simulink subsystem "AllControllers"  (R2020b)
settings: Solver=VariableStepAuto  StartTime=0.0  StopTime=10.0  RelTol=1e-3
values from neighbouring files (symbols this model uses):
  A = d_sys.A    [MPC_Init.m]    (also in init.m = [a11 a12 0 0;     a21 a22 0 0;     0 1 0 0;     v ls v 0])
  B = d_sys.B    [MPC_Init.m]    (also in init.m = [2*cf/(m*v) 0; 2*lf*cf/iz 0; 0 -v ;0  0])
  C = d_sys.C    [MPC_Init.m]    (also in init.m = [0 0 1 0; 0 0 0 1])
  K = place(A,B,kp)    [init.m]
  L = place(A',C',kl)    [init.m]
  Ts = 0.1    [MPC_Init.m]
undefined symbols (not defined in the file or in its folder): DiscIntNeverNeededParam, lkasubsystem_1_data, PredictionHorizon
libraries: mpclib x1, simulink x1, mpcadaslib x1, pid_lib x1
settings Model: Creator=Stage  LastModifiedBy=Stage

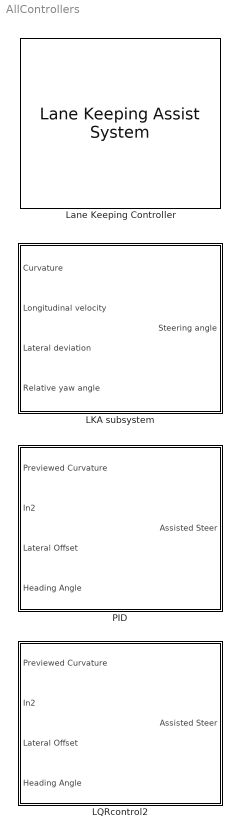
== system AllControllers ==
  LKA subsystem : Subsystem
  LQRcontrol2 : Subsystem
  Lane Keeping Controller : mpcadaslib/Lane Keeping Assist System  ModelType=Use vehicle parameters  VehicleMass=m  VehicleYawInertia=Iz  LengthToFront=lf  LengthToRear=lr  FrontTireStiffness=Cf  RearTireStiffness=Cr  EgoModelMatrixA=[-4.4021 ,-12.4603;1.3913,-5.1868]  EgoModelMatrixB=[24.1270;15.8609]  EgoModelMatrixC=[1,0;0,1]  InitialLongVel=v0_ego  TransportLag=0  MinSteering=-0.5  umin_ext=off  MaxSteering=0.5  umax_ext=off  Ts=Ts  PredictionHorizon=PredictionHorizon  ControllerBehavior=0.200  suboptimal=off  maxiter=10  datatypeopt=single  optmode=off  trackmode=off
      settings: SourceProductBaseCode=MP
  PID : Subsystem

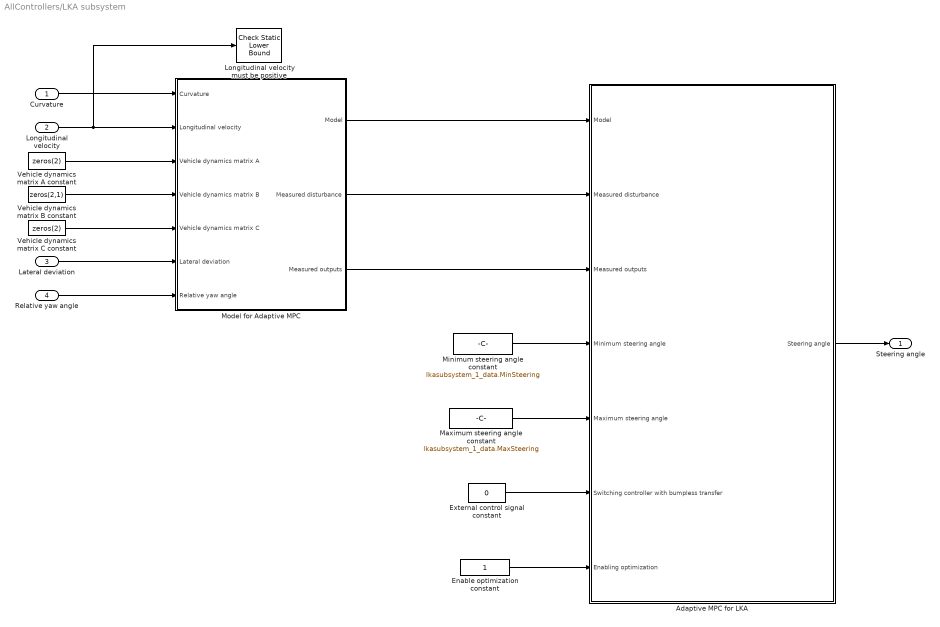
== system AllControllers/LKA subsystem ==
  Curvature : Inport
  Longitudinal velocity : Inport  Port=2
  Lateral deviation : Inport  Port=3
  Relative yaw angle : Inport  Port=4
  Adaptive MPC for LKA : Subsystem
  Enable optimization constant : Constant  OutDataTypeStr=lkasubsystem_1_data.DataType
  External control signal constant : Constant  Value=0  OutDataTypeStr=lkasubsystem_1_data.DataType
  Longitudinal velocity must be positive : simulink/Model Verification/Check Static  Lower Bound  Description=0 < u  min=0  min_included=off  enabled=on  stopWhenAssertionFail=on  export=off  icon=graphic
  Maximum steering angle constant : Constant  Value=lkasubsystem_1_data.MaxSteering  OutDataTypeStr=lkasubsystem_1_data.DataType
  Minimum steering angle constant : Constant  Value=lkasubsystem_1_data.MinSteering  OutDataTypeStr=lkasubsystem_1_data.DataType
  Model for Adaptive MPC : Subsystem
  Vehicle dynamics matrix A constant : Constant  Value=zeros(2)  OutDataTypeStr=lkasubsystem_1_data.DataType
  Vehicle dynamics matrix B constant : Constant  Value=zeros(2,1)  OutDataTypeStr=lkasubsystem_1_data.DataType
  Vehicle dynamics matrix C constant : Constant  Value=zeros(2)  OutDataTypeStr=lkasubsystem_1_data.DataType
  Steering angle : Outport  VectorParamsAs1DForOutWhenUnconnected=off
  wires:
  Longitudinal velocity/1 -> Longitudinal velocity must be positive/1, Model for Adaptive MPC/2(Longitudinal velocity)
  Curvature/1 -> Model for Adaptive MPC/1(Curvature)
  Model for Adaptive MPC/1(Model) -> Adaptive MPC for LKA/1(Model)
  Adaptive MPC for LKA/1(Steering angle) -> Steering angle/1
  Model for Adaptive MPC/2(Measured disturbance) -> Adaptive MPC for LKA/2(Measured disturbance)
  Enable optimization constant/1 -> Adaptive MPC for LKA/7(Enabling optimization)
  External control signal constant/1 -> Adaptive MPC for LKA/6(Switching controller with bumpless transfer)
  Minimum steering angle constant/1 -> Adaptive MPC for LKA/4(Minimum steering angle)
  Maximum steering angle constant/1 -> Adaptive MPC for LKA/5(Maximum steering angle)
  Model for Adaptive MPC/3(Measured outputs) -> Adaptive MPC for LKA/3(Measured outputs)
  Lateral deviation/1 -> Model for Adaptive MPC/6(Lateral deviation)
  Relative yaw angle/1 -> Model for Adaptive MPC/7(Relative yaw angle)
  Vehicle dynamics matrix A constant/1 -> Model for Adaptive MPC/3(Vehicle dynamics matrix A)
  Vehicle dynamics matrix B constant/1 -> Model for Adaptive MPC/4(Vehicle dynamics matrix B)
  Vehicle dynamics matrix C constant/1 -> Model for Adaptive MPC/5(Vehicle dynamics matrix C)

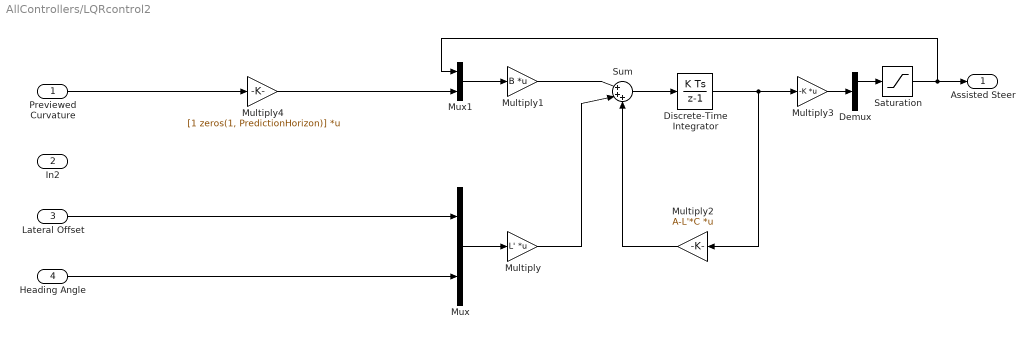
== system AllControllers/LQRcontrol2 ==
  Previewed Curvature : Inport
  In2 : Inport  Port=2
  Lateral Offset : Inport  Port=3
  Heading Angle : Inport  Port=4
  Demux : Demux  Outputs=2
  Discrete-Time Integrator : DiscreteIntegrator  SampleTime=-1  ICPrevOutput=DiscIntNeverNeededParam  ICPrevScaledInput=DiscIntNeverNeededParam
  Multiply : Gain  Gain=L'  Multiplication=Matrix(K*u) (u vector)
  Multiply1 : Gain  Gain=B  Multiplication=Matrix(K*u) (u vector)
  Multiply2 : Gain  Gain=A-L'*C  Multiplication=Matrix(K*u) (u vector)
  Multiply3 : Gain  Gain=-K  Multiplication=Matrix(K*u) (u vector)
  Multiply4 : Gain  Gain=[1 zeros(1, PredictionHorizon)]  Multiplication=Matrix(K*u) (u vector)
  Mux : Mux  Inputs=2
  Mux1 : Mux  Inputs=2
  Saturation : Saturate  UpperLimit=0.2  LowerLimit=-0.2
  Sum : Sum  Inputs=|+++
  Assisted Steer : Outport
  wires:
  Heading Angle/1 -> Mux/2
  Lateral Offset/1 -> Mux/1
  Mux/1 -> Multiply/1
  Demux/1 -> Saturation/1
  Previewed Curvature/1 -> Multiply4/1
  Multiply4/1 -> Mux1/2
  Mux1/1 -> Multiply1/1
  Multiply1/1 -> Sum/1
  Multiply/1 -> Sum/2
  Sum/1 -> Discrete-Time Integrator/1
  Discrete-Time Integrator/1 -> Multiply2/1, Multiply3/1
  Multiply2/1 -> Sum/3
  Multiply3/1 -> Demux/1
  Saturation/1 -> Assisted Steer/1, Mux1/1

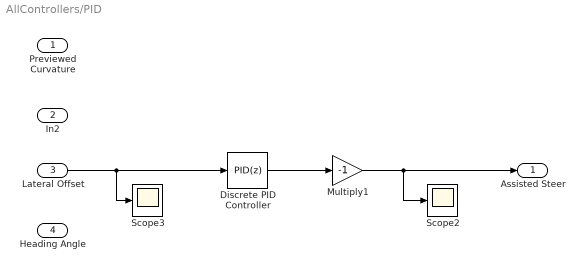
== system AllControllers/PID ==
  Previewed Curvature : Inport
  In2 : Inport  Port=2
  Lateral Offset : Inport  Port=3
  Heading Angle : Inport  Port=4
  Discrete PID Controller : pid_lib/PID Controller  Controller=PID  Form=Parallel  TimeDomain=Discrete-time  UseExternalTs=off  SampleTime=-1  IntegratorMethod=Forward Euler  FilterMethod=Forward Euler  ControllerParametersSource=internal  P=0.5  I=0.05  D=0.08  UseFilter=off  N=100  TunerSelectOption=Transfer Function Based (PID Tuner App)  InitialConditionSource=internal  InitialConditionForIntegrator=0  InitialConditionForFilter=0  DifferentiatorICPrevScaledInput=0  ExternalReset=none  TrackingMode=off  Kt=1  LimitOutput=off  SatLimitsSource=internal  UpperSaturationLimit=inf  LowerSaturationLimit=-inf  LinearizeAsGain=off  AntiWindupMode=none  Kb=1  POutMin=[]  POutMax=[]  IOutMin=[]  IOutMax=[]  DOutMin=[]  DOutMax=[]  NOutMin=[]  NOutMax=[]  SumOutMin=[]  SumOutMax=[]  SaturationOutMin=[]  SaturationOutMax=[]  PParamMin=[]  PParamMax=[]  IParamMin=[]  IParamMax=[]  DParamMin=[]  DParamMax=[]  NParamMin=[]  NParamMax=[]  KbParamMin=[]  KbParamMax=[]  KtParamMin=[]  KtParamMax=[]  KbOutMin=[]  KbOutMax=[]  KtOutMin=[]  KtOutMax=[]  IntegratorOutMin=[]  IntegratorOutMax=[]  FilterOutMin=[]  FilterOutMax=[]  SumI1OutMin=[]  SumI1OutMax=[]  SumI2OutMin=[]  SumI2OutMax=[]  SumI3OutMin=[]  SumI3OutMax=[]  SumI4OutMin=[]  SumI4OutMax=[]  SumDOutMin=[]  SumDOutMax=[]  DifferentiatorOutMin=[]  DifferentiatorOutMax=[]  FilterDiffOutCoefMin=[]  FilterDiffOutCoefMax=[]  ReciprocalOutMin=[]  ReciprocalOutMax=[]  SumDenOutMin=[]  SumDenOutMax=[]  SumNumOutMin=[]  SumNumOutMax=[]  DivideOutMin=[]  DivideOutMax=[]  UdiffTsProdOutMin=[]  UdiffTsProdOutMax=[]  NTsProdOutMin=[]  NTsProdOutMax=[]  UintegralTsProdOutMin=[]  UintegralTsProdOutMax=[]  UngainTsProdOutMin=[]  UngainTsProdOutMax=[]  IntegratorContinuousStateAttributes=''  IntegratorStateMustResolveToSignalObject=off  IntegratorRTWStateStorageClass=Auto  FilterContinuousStateAttributes=''  FilterStateMustResolveToSignalObject=off  FilterRTWStateStorageClass=Auto  ParallelPVariant=InternalParameters  IdealPVariant=Disabled  IVariant=InternalParameters  DVariant=InternalParameters  IntegratorVariant=Discrete  SatVariant=Disabled  AWVariant=Passthrough  PCopyVariant=Disabled  TRVariant=Disabled  FdbkBlocksVariant=Forward  IdealPFdbkVariant=Disabled  SatFdbkVariant=Disabled  DerivativeFilterVariant=Differentiator  NVariant=Passthrough  NCopyVariant=Disabled_SignalSpec  FilterICVariant=InternalICsDifferentiator  IntegratorICVariant=InternalICs  ExternalResetVariant=Disabled  TRSumVariant=Passthrough  SumFdbkVariant=Disabled  SumVariant=Sum_PID  TsampFilterVariant=InternalTs  TsampNgainVariant=Passthrough  TsampIntegralVariant=Passthrough  ExternalSaturationOutDataTypeStr=Inherit: Same as second input
  Multiply1 : Gain  Gain=-1
  Scope2 : Scope
  Scope3 : Scope
  Assisted Steer : Outport
  wires:
  Lateral Offset/1 -> Scope3/1, Discrete PID Controller/1
  Discrete PID Controller/1 -> Multiply1/1
  Multiply1/1 -> Assisted Steer/1, Scope2/1

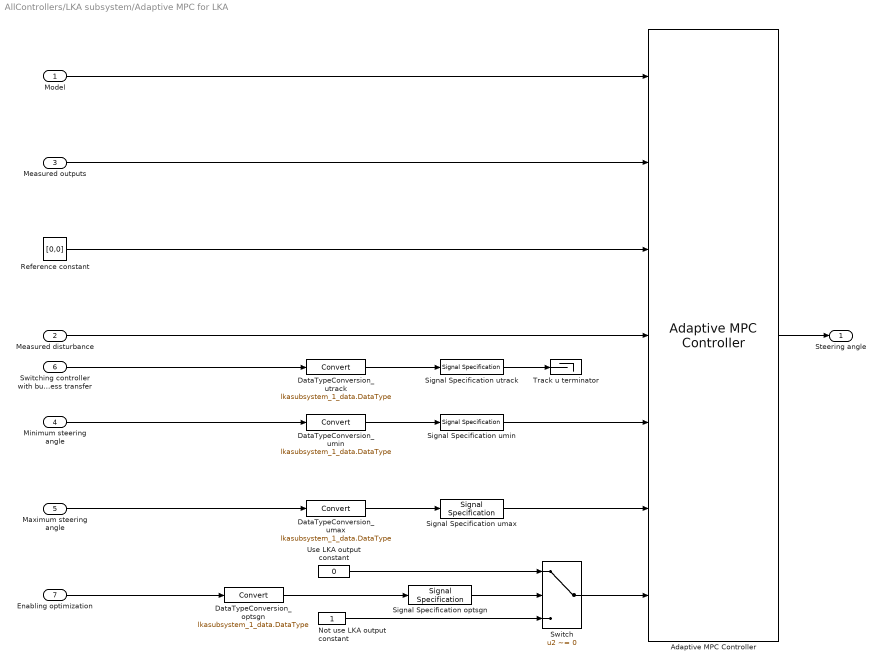
== system AllControllers/LKA subsystem/Adaptive MPC for LKA ==
  Model : Inport
  Measured disturbance : Inport  Port=2
  Measured outputs : Inport  Port=3
  Minimum steering angle : Inport  Port=4
  Maximum steering angle : Inport  Port=5
  Switching controller with bumpless transfer : Inport  Port=6
  Enabling optimization : Inport  Port=7
  Adaptive MPC Controller : mpclib/Adaptive MPC Controller  SCDEnableBlockLinearizationSpecification=on  mpcobj=lkasubsystem_1_data.Controller  enable_value=0  updateMPCinCallerWorkspace=off  md_inport=on  mv_inport=off  uref_inport=off  return_cost=off  return_mvseq=off  return_qpstatus=off  return_xseq=off  return_state=off  return_ovseq=off  state_inport=off  isltv_plant=off  umin_inport=on  umax_inport=on  ymin_inport=off  ymax_inport=off  cc_inport=off  ywt_inport=off  uwt_inport=off  duwt_inport=off  rhoeps_inport=off  pm_inport=off  MaximumP=10  HorizonChoice=FixedHorizon  BlockDataType=single  SampleTimeInherited=off  switch_inport=on
      settings: SourceProductName=Model Predictive Control Toolbox
  DataTypeConversion_optsgn : DataTypeConversion  OutDataTypeStr=lkasubsystem_1_data.DataType
  DataTypeConversion_umax : DataTypeConversion  OutDataTypeStr=lkasubsystem_1_data.DataType
  DataTypeConversion_umin : DataTypeConversion  OutDataTypeStr=lkasubsystem_1_data.DataType
  DataTypeConversion_utrack : DataTypeConversion  OutDataTypeStr=lkasubsystem_1_data.DataType
  Not use LKA output constant : Constant  OutDataTypeStr=lkasubsystem_1_data.DataType
  Reference constant : Constant  Value=[0,0]  VectorParams1D=off  OutDataTypeStr=lkasubsystem_1_data.DataType
  Signal Specification optsgn : SignalSpecification  Dimensions=1
  Signal Specification umax : SignalSpecification  Dimensions=1
  Signal Specification umin : SignalSpecification  Dimensions=1
  Signal Specification utrack : SignalSpecification  Dimensions=1
  Switch : Switch  Criteria=u2 ~= 0
  Track u terminator : Terminator
  Use LKA output constant : Constant  Value=0  OutDataTypeStr=lkasubsystem_1_data.DataType
  Steering angle : Outport  VectorParamsAs1DForOutWhenUnconnected=off
  wires:
  Not use LKA output constant/1 -> Switch/3
  DataTypeConversion_umin/1 -> Signal Specification umin/1
  Measured disturbance/1 -> Adaptive MPC Controller/4
  Switching controller with bumpless transfer/1 -> DataTypeConversion_utrack/1
  DataTypeConversion_umax/1 -> Signal Specification umax/1
  Use LKA output constant/1 -> Switch/1
  Adaptive MPC Controller/1 -> Steering angle/1
  DataTypeConversion_utrack/1 -> Signal Specification utrack/1
  DataTypeConversion_optsgn/1 -> Signal Specification optsgn/1
  Signal Specification optsgn/1 -> Switch/2
  Reference constant/1 -> Adaptive MPC Controller/3
  Switch/1 -> Adaptive MPC Controller/7
  Minimum steering angle/1 -> DataTypeConversion_umin/1
  Model/1 -> Adaptive MPC Controller/1
  Signal Specification umin/1 -> Adaptive MPC Controller/5
  Maximum steering angle/1 -> DataTypeConversion_umax/1
  Enabling optimization/1 -> DataTypeConversion_optsgn/1
  Measured outputs/1 -> Adaptive MPC Controller/2
  Signal Specification umax/1 -> Adaptive MPC Controller/6
  Signal Specification utrack/1 -> Track u terminator/1

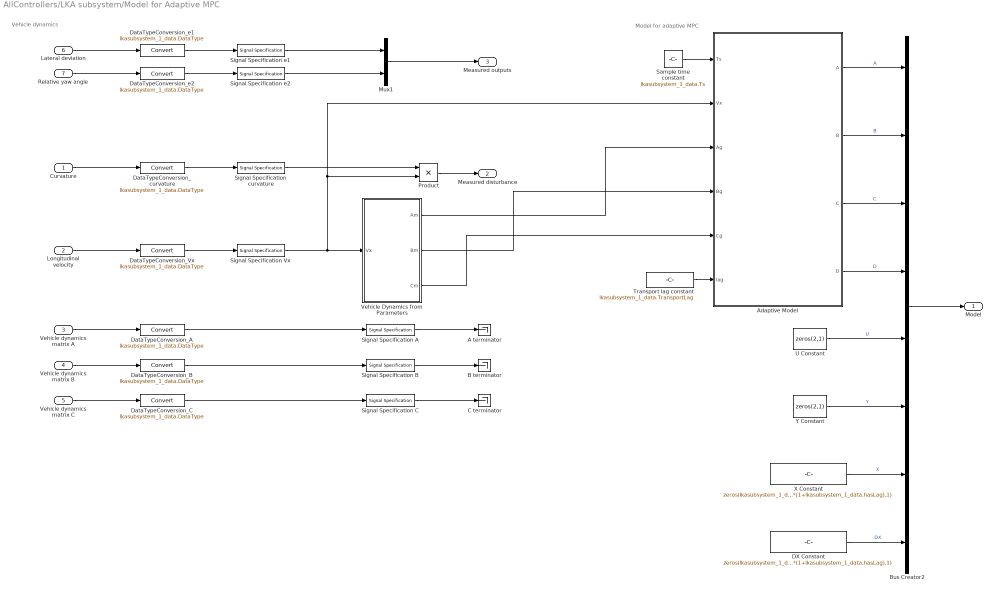
== system AllControllers/LKA subsystem/Model for Adaptive MPC ==
  note: Model for adaptive MPC
  note: Vehicle dynamics
  Curvature : Inport
  Longitudinal velocity : Inport  Port=2
  Vehicle dynamics matrix A : Inport  Port=3
  Vehicle dynamics matrix B : Inport  Port=4
  Vehicle dynamics matrix C : Inport  Port=5
  Lateral deviation : Inport  Port=6
  Relative yaw angle : Inport  Port=7
  A terminator : Terminator
  Adaptive Model : MATLAB Function  TreatAsAtomicUnit=on
  B terminator : Terminator
  Bus Creator2 : BusCreator  Inputs=8
  C terminator : Terminator
  DX Constant : Constant  Value=zeros(lkasubsystem_1_data.NumEgoStates+2*(1+lkasubsystem_1_data.hasLag),1)  VectorParams1D=off  OutDataTypeStr=lkasubsystem_1_data.DataType
  DataTypeConversion_A : DataTypeConversion  OutDataTypeStr=lkasubsystem_1_data.DataType
  DataTypeConversion_B : DataTypeConversion  OutDataTypeStr=lkasubsystem_1_data.DataType
  DataTypeConversion_C : DataTypeConversion  OutDataTypeStr=lkasubsystem_1_data.DataType
  DataTypeConversion_Vx : DataTypeConversion  OutDataTypeStr=lkasubsystem_1_data.DataType
  DataTypeConversion_curvature : DataTypeConversion  OutDataTypeStr=lkasubsystem_1_data.DataType
  DataTypeConversion_e1 : DataTypeConversion  OutDataTypeStr=lkasubsystem_1_data.DataType
  DataTypeConversion_e2 : DataTypeConversion  OutDataTypeStr=lkasubsystem_1_data.DataType
  Mux1 : Mux  Inputs=[1 1]
  Product : Product
  Sample time constant : Constant  Value=lkasubsystem_1_data.Ts  OutDataTypeStr=lkasubsystem_1_data.DataType
  Signal Specification A : SignalSpecification
  Signal Specification B : SignalSpecification
  Signal Specification C : SignalSpecification
  Signal Specification Vx : SignalSpecification  Dimensions=1
  Signal Specification curvature : SignalSpecification
  Signal Specification e1 : SignalSpecification  Dimensions=1
  Signal Specification e2 : SignalSpecification  Dimensions=1
  Transport lag constant : Constant  Value=lkasubsystem_1_data.TransportLag  OutDataTypeStr=lkasubsystem_1_data.DataType
  U Constant : Constant  Value=zeros(2,1)  VectorParams1D=off  OutDataTypeStr=lkasubsystem_1_data.DataType
  Vehicle Dynamics from Parameters : Subsystem
  X Constant : Constant  Value=zeros(lkasubsystem_1_data.NumEgoStates+2*(1+lkasubsystem_1_data.hasLag),1)  VectorParams1D=off  OutDataTypeStr=lkasubsystem_1_data.DataType
  Y Constant : Constant  Value=zeros(2,1)  VectorParams1D=off  OutDataTypeStr=lkasubsystem_1_data.DataType
  Model : Outport  VectorParamsAs1DForOutWhenUnconnected=off
  Measured disturbance : Outport  Port=2  VectorParamsAs1DForOutWhenUnconnected=off
  Measured outputs : Outport  Port=3  VectorParamsAs1DForOutWhenUnconnected=off
  wires:
  Sample time constant/1 -> Adaptive Model/1(Ts)
  Bus Creator2/1 -> Model/1
  Curvature/1 -> DataTypeConversion_curvature/1
  X Constant/1 -> Bus Creator2/7  "X"
  DX Constant/1 -> Bus Creator2/8  "DX"
  Vehicle dynamics matrix B/1 -> DataTypeConversion_B/1
  Vehicle dynamics matrix C/1 -> DataTypeConversion_C/1
  Vehicle dynamics matrix A/1 -> DataTypeConversion_A/1
  Longitudinal velocity/1 -> DataTypeConversion_Vx/1
  Product/1 -> Measured disturbance/1
  DataTypeConversion_Vx/1 -> Signal Specification Vx/1
  Signal Specification Vx/1 -> Adaptive Model/2(Vx), Product/2, Vehicle Dynamics from Parameters/1(Vx)
  DataTypeConversion_curvature/1 -> Signal Specification curvature/1
  DataTypeConversion_A/1 -> Signal Specification A/1
  DataTypeConversion_B/1 -> Signal Specification B/1
  DataTypeConversion_C/1 -> Signal Specification C/1
  Signal Specification curvature/1 -> Product/1
  Lateral deviation/1 -> DataTypeConversion_e1/1
  Signal Specification e1/1 -> Mux1/1
  DataTypeConversion_e2/1 -> Signal Specification e2/1
  Relative yaw angle/1 -> DataTypeConversion_e2/1
  Signal Specification e2/1 -> Mux1/2
  DataTypeConversion_e1/1 -> Signal Specification e1/1
  Mux1/1 -> Measured outputs/1
  Adaptive Model/1(A) -> Bus Creator2/1  "A"
  Adaptive Model/2(B) -> Bus Creator2/2  "B"
  Adaptive Model/3(C) -> Bus Creator2/3  "C"
  Adaptive Model/4(D) -> Bus Creator2/4  "D"
  U Constant/1 -> Bus Creator2/5  "U"
  Y Constant/1 -> Bus Creator2/6  "Y"
  Transport lag constant/1 -> Adaptive Model/6(lag)
  Signal Specification A/1 -> A terminator/1
  Signal Specification B/1 -> B terminator/1
  Signal Specification C/1 -> C terminator/1
  Vehicle Dynamics from Parameters/1(Am) -> Adaptive Model/3(Ag)
  Vehicle Dynamics from Parameters/2(Bm) -> Adaptive Model/4(Bg)
  Vehicle Dynamics from Parameters/3(Cm) -> Adaptive Model/5(Cg)

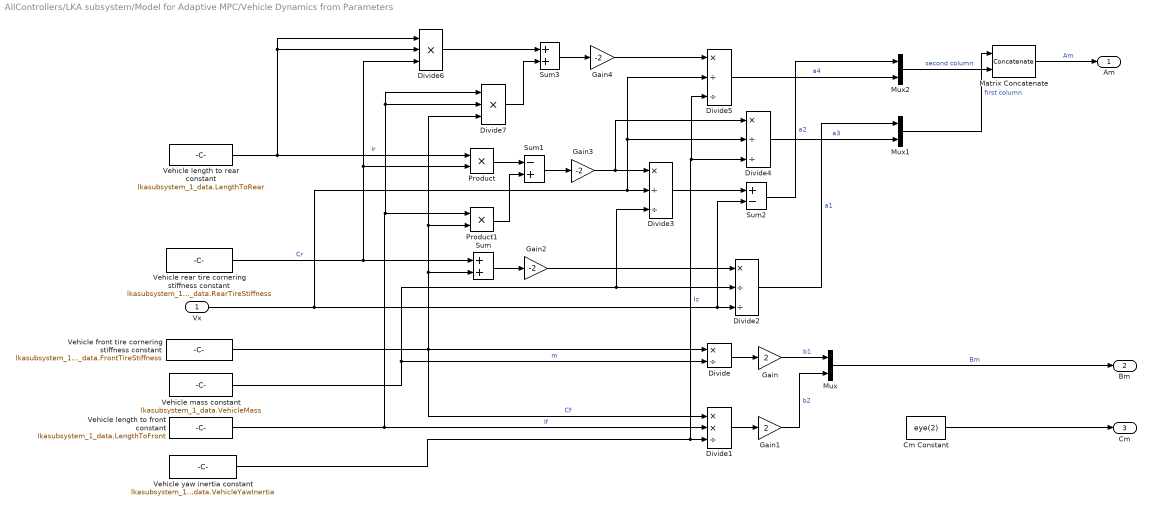
== system AllControllers/LKA subsystem/Model for Adaptive MPC/Vehicle Dynamics from Parameters ==
  Vx : Inport
  Cm Constant : Constant  Value=eye(2)  OutDataTypeStr=lkasubsystem_1_data.DataType
  Divide : Product  Inputs=*/
  Divide1 : Product  Inputs=**/
  Divide{2..5} (4 alike) : Product  Inputs=*//
  Divide6 : Product  Inputs=***
  Divide7 : Product  Inputs=***
  Gain : Gain  Gain=2
  Gain1 : Gain  Gain=2
  Gain2 : Gain  Gain=-2
  Gain3 : Gain  Gain=-2
  Gain4 : Gain  Gain=-2
  Matrix Concatenate : Concatenate  Mode=Multidimensional array  ConcatenateDimension=2
  Mux : Mux  Inputs=[1 1]
  Mux1 : Mux  Inputs=[1 1]
  Mux2 : Mux  Inputs=[1 1]
  Product : Product
  Product1 : Product
  Sum : Sum
  Sum1 : Sum  Inputs=-+
  Sum2 : Sum  Inputs=+-
  Sum3 : Sum
  Vehicle front tire cornering stiffness constant : Constant  Value=lkasubsystem_1_data.FrontTireStiffness  OutDataTypeStr=lkasubsystem_1_data.DataType
  Vehicle length to front constant : Constant  Value=lkasubsystem_1_data.LengthToFront  OutDataTypeStr=lkasubsystem_1_data.DataType
  Vehicle length to rear constant : Constant  Value=lkasubsystem_1_data.LengthToRear  OutDataTypeStr=lkasubsystem_1_data.DataType
  Vehicle mass constant : Constant  Value=lkasubsystem_1_data.VehicleMass  OutDataTypeStr=lkasubsystem_1_data.DataType
  Vehicle rear tire cornering stiffness constant : Constant  Value=lkasubsystem_1_data.RearTireStiffness  OutDataTypeStr=lkasubsystem_1_data.DataType
  Vehicle yaw inertia constant : Constant  Value=lkasubsystem_1_data.VehicleYawInertia  OutDataTypeStr=lkasubsystem_1_data.DataType
  Am : Outport  VectorParamsAs1DForOutWhenUnconnected=off
  Bm : Outport  Port=2  VectorParamsAs1DForOutWhenUnconnected=off
  Cm : Outport  Port=3  VectorParamsAs1DForOutWhenUnconnected=off
  wires:
  Vehicle front tire cornering stiffness constant/1 -> Divide1/1, Divide/1, Divide7/3, Product1/2, Sum/2  "Cf"
  Vehicle length to front constant/1 -> Divide7/1, Divide7/2, Product1/1, Divide1/2  "lf"
  Vehicle mass constant/1 -> Divide/2, Divide3/3, Divide2/2  "m"
  Divide/1 -> Gain/1
  Product/1 -> Sum1/1
  Vehicle length to rear constant/1 -> Divide6/2, Divide6/1, Product/1  "lr"
  Gain2/1 -> Divide2/1
  Vehicle yaw inertia constant/1 -> Divide5/3, Divide4/3, Divide1/3  "Iz"
  Gain1/1 -> Mux/2  "b2"
  Vehicle rear tire cornering stiffness constant/1 -> Divide6/3, Product/2, Sum/1  "Cr"
  Divide5/1 -> Mux2/2  "a4"
  Gain4/1 -> Divide5/1
  Sum1/1 -> Gain3/1
  Sum/1 -> Gain2/1
  Sum3/1 -> Gain4/1
  Gain3/1 -> Divide3/1, Divide4/1
  Vx/1 -> Divide3/2, Divide5/2, Divide4/2, Sum2/2, Divide2/3
  Sum2/1 -> Mux2/1  "a2"
  Divide7/1 -> Sum3/2
  Divide2/1 -> Mux1/1  "a1"
  Mux1/1 -> Matrix Concatenate/1  "first column"
  Divide4/1 -> Mux1/2  "a3"
  Divide3/1 -> Sum2/1
  Matrix Concatenate/1 -> Am/1  "Am"
  Mux2/1 -> Matrix Concatenate/2  "second column"
  Product1/1 -> Sum1/2
  Divide6/1 -> Sum3/1
  Divide1/1 -> Gain1/1
  Gain/1 -> Mux/1  "b1"
  Mux/1 -> Bm/1  "Bm"
  Cm Constant/1 -> Cm/1

== matlab function AllControllers/LKA subsystem/Model for Adaptive MPC/Adaptive Model ==
  data: A output; B output; C output; D output size=[2,2]; Ts input size=1; Vx input size=1; Ag input; Bg input; Cg input; lag input
function [A,B,C,D] = getAdaptiveMPCModel(Ts,Vx,Ag,Bg,Cg,lag)

% Get discrete state-space model for Adaptive MPC with sample time Ts.
% Called by the 'Lane Keeping Assist System' Block.

% Inputs:
%   Ts:               mask variable for sample time
%   Vx:               mask inport for longitudinal velocity
%   Ag,Bg,Cg:         continuous or discrete vehicle model
%   lag:              lumped lag in the model
% Outputs:
%   A,B,C,D:          discrete time model for adaptive MPC

%   Author: Meng Xia, Rong Chen
%   Copyright 2017-2018 The MathWorks, Inc.

% Discrete MPC model
[A,B,C,D] = lkablock_utilGetDTModelNoLagForMPC(Ts,Vx,Ag,Bg,Cg);
